simulink model "semi_solarwind"  (R2023b)
settings: Solver=VariableStepAuto  StartTime=0.0  StopTime=5  RelTol=1e-3
undefined symbols (not defined in the file): D1, Delta, Ion, Lithium
libraries: spsSeriesRLCBranchLib x26, spsVoltageMeasurementLib x9, spsDiodeLib x8, dspsrcs4 x8, spsCurrentMeasurementLib x5, spsThreePhaseVIMeasurementLib x5, spsMosfetLib x4, spsPWMGeneratorDCDCLib x4, spsPVArrayLib x4, spsThreePhaseTransformerTwoWindingsLib x3, spsThreePhaseParallelRLCLoadLib x3, spsThreePhaseSeriesRLCBranchLib x3
(part 2 of 2)

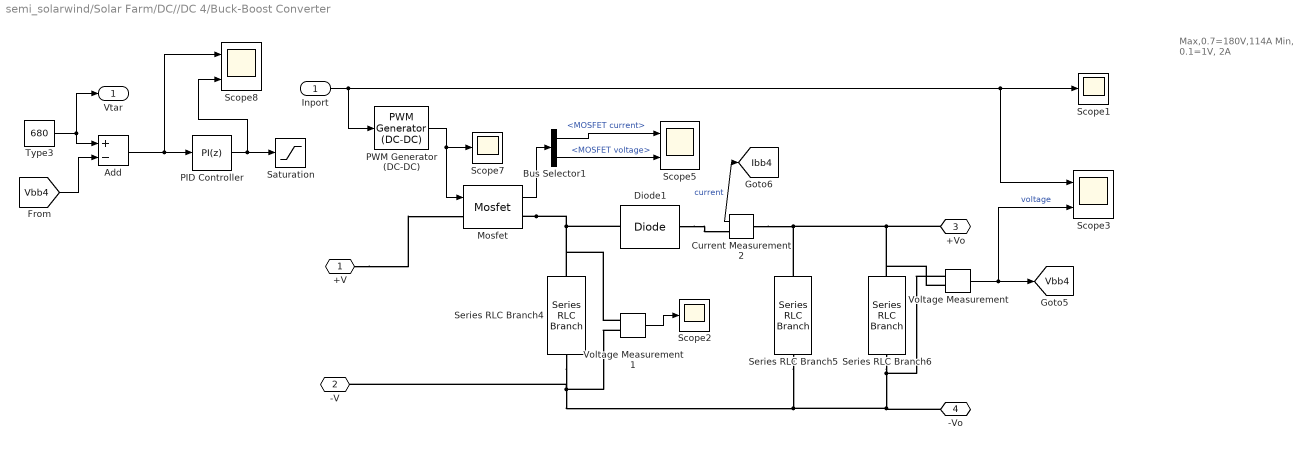
== system semi_solarwind/Solar Farm/DC//DC 4/Buck-Boost Converter ==
  note: Max,0.7=180V,114A
      | Min, 0.1=1V, 2A
  Inport : Inport
  Add : Sum  Inputs=+-
  Bus Selector1 : BusSelector  OutputSignals=MOSFET current,MOSFET voltage
  Current Measurement2 : spsCurrentMeasurementLib/Current Measurement  PhasorSimulation=off  OutputType=Complex  PSBequivalent=0
  Diode1 : spsDiodeLib/Diode  Ron=0.001  Lon=0  Vf=0.8  IC=0  UseSnubber=0  Rs=500  Cs=250e-9  Measurements=off
  Mosfet : spsMosfetLib/Mosfet  Ron=0.1  Lon=0  Rd=0.01  Vfd=0  IC=0  Rs=1e5  Cs=inf  Measurements=on
  PID Controller : slpidlib/PID Controller  Controller=PI  Form=Parallel  TimeDomain=Discrete-time  UseExternalTs=off  SampleTime=-1  IntegratorMethod=Forward Euler  FilterMethod=Forward Euler  ControllerParametersSource=internal  P=0.448206848938492  I=8.01083955194228  UseKiTs=off  D=0  N=100  UseFilter=on  TunerSelectOption=Transfer Function Based (PID Tuner App)  InitialConditionSource=internal  InitialConditionForIntegrator=0  InitialConditionForFilter=0  DifferentiatorICPrevScaledInput=0  ExternalReset=none  TrackingMode=off  Kt=1  LimitOutput=on  SatLimitsSource=internal  UpperSaturationLimit=0.8  LowerSaturationLimit=0  LinearizeAsGain=off  AntiWindupMode=none  Kb=1  LimitIntegrator=on  UpperIntegratorSaturationLimit=0.8  LowerIntegratorSaturationLimit=0  POutMin=[]  POutMax=[]  IOutMin=[]  IOutMax=[]  DOutMin=[]  DOutMax=[]  NOutMin=[]  NOutMax=[]  SumOutMin=[]  SumOutMax=[]  SaturationOutMin=[]  SaturationOutMax=[]  PParamMin=[]  PParamMax=[]  IParamMin=[]  IParamMax=[]  DParamMin=[]  DParamMax=[]  NParamMin=[]  NParamMax=[]  KbParamMin=[]  KbParamMax=[]  KtParamMin=[]  KtParamMax=[]  KbOutMin=[]  KbOutMax=[]  KtOutMin=[]  KtOutMax=[]  IntegratorOutMin=[]  IntegratorOutMax=[]  FilterOutMin=[]  FilterOutMax=[]  SumI1OutMin=[]  SumI1OutMax=[]  SumI2OutMin=[]  SumI2OutMax=[]  SumI3OutMin=[]  SumI3OutMax=[]  SumI4OutMin=[]  SumI4OutMax=[]  SumDOutMin=[]  SumDOutMax=[]  DifferentiatorOutMin=[]  DifferentiatorOutMax=[]  FilterDiffOutCoefMin=[]  FilterDiffOutCoefMax=[]  ReciprocalOutMin=[]  ReciprocalOutMax=[]  SumDenOutMin=[]  SumDenOutMax=[]  SumNumOutMin=[]  SumNumOutMax=[]  DivideOutMin=[]  DivideOutMax=[]  UdiffTsProdOutMin=[]  UdiffTsProdOutMax=[]  NTsProdOutMin=[]  NTsProdOutMax=[]  UintegralTsProdOutMin=[]  UintegralTsProdOutMax=[]  UngainTsProdOutMin=[]  UngainTsProdOutMax=[]  ClampingZeroOutDataTypeStr=Inherit: Inherit via back propagation  ClampingZeroOutMin=[]  ClampingZeroOutMax=[]  FilterDenConstantOutDataTypeStr=Inherit: Inherit via back propagation  FilterDenConstantOutMin=[]  FilterDenConstantOutMax=[]  PCopyOutDataTypeStr=Inherit: Inherit via back propagation  PCopyOutMin=[]  PCopyOutMax=[]  NCopyOutDataTypeStr=Inherit: Inherit via back propagation  NCopyOutMin=[]  NCopyOutMax=[]  IntegratorContinuousStateAttributes=''  IntegratorStateMustResolveToSignalObject=off  IntegratorRTWStateStorageClass=Auto  FilterContinuousStateAttributes=''  FilterStateMustResolveToSignalObject=off  FilterRTWStateStorageClass=Auto  ParallelPVariant=InternalParameters  IdealPVariant=Disabled  IVariant=InternalParameters  DVariant=Disabled  IntegratorVariant=Discrete  SatVariant=Enabled  AWVariant=Passthrough  PCopyVariant=Disabled  TRVariant=Disabled  FdbkBlocksVariant=Forward  IdealPFdbkVariant=Disabled  SatFdbkVariant=Disabled  DerivativeFilterVariant=Disabled  NVariant=Disabled  NCopyVariant=Disabled_SignalSpec  FilterICVariant=Disabled  IntegratorICVariant=InternalICs  ExternalResetVariant=Disabled  TRSumVariant=Passthrough  SumFdbkVariant=Disabled  SumVariant=Sum_PI  TsampFilterVariant=InternalTs  TsampNgainVariant=Passthrough  TsampIntegralVariant=Disabled_SignalSpec  ExternalSaturationOutDataTypeStr=Inherit: Same as second input
  PWM Generator (DC-DC) : spsPWMGeneratorDCDCLib/PWM Generator (DC-DC)  Fsw=900  Ts=0
  Saturation : Saturate  UpperLimit=0.8  LowerLimit=0
  Scope1 : Scope
  Scope2 : Scope
  Scope3 : Scope  NumInputPorts=2
  Scope5 : Scope  NumInputPorts=2
  Scope7 : Scope
  Scope8 : Scope  NumInputPorts=2
  Series RLC Branch4 : spsSeriesRLCBranchLib/Series RLC Branch  LConnTagsString=__new0  RConnTagsString=__new0  BranchType=L  Resistance=1  Inductance=1e-3  SetiL0=off  InitialCurrent=0  Capacitance=1e-6  Setx0=off  InitialVoltage=0  Measurements=None
  Series RLC Branch5 : spsSeriesRLCBranchLib/Series RLC Branch  LConnTagsString=__new0  RConnTagsString=__new0  BranchType=C  Resistance=1  Inductance=1e-3  SetiL0=off  InitialCurrent=0  Capacitance=1e-2  Setx0=off  InitialVoltage=0  Measurements=None
  Series RLC Branch6 : spsSeriesRLCBranchLib/Series RLC Branch  LConnTagsString=__new0  RConnTagsString=__new0  BranchType=R  Resistance=50  Inductance=1e-3  SetiL0=off  InitialCurrent=0  Capacitance=1e-6  Setx0=off  InitialVoltage=0  Measurements=None
  Type3 : Constant  Value=680  SampleTime=0
  Voltage Measurement : spsVoltageMeasurementLib/Voltage Measurement  PhasorSimulation=off  OutputType=Complex  PSBequivalent=0
  Voltage Measurement1 : spsVoltageMeasurementLib/Voltage Measurement  PhasorSimulation=off  OutputType=Complex  PSBequivalent=0
  +V : PMIOPort  Side=Left
  -V : PMIOPort  Port=2  Side=Left
  +Vo : PMIOPort  Port=3  Side=Right
  -Vo : PMIOPort  Port=4  Side=Right
  Vtar : Outport
  tag scope: Ibb4=global, Vbb4=global
  wires:
  [Vbb4] -> Add/2
  Voltage Measurement/1 -> Scope3/2, [Vbb4]  "voltage"
  Bus Selector1/1 -> Scope5/1  "<MOSFET current>"
  Voltage Measurement1/1 -> Scope2/1
  Bus Selector1/2 -> Scope5/2  "<MOSFET voltage>"
  PID Controller/1 -> Scope8/2, Saturation/1
  Add/1 -> Scope8/1, PID Controller/1
  Current Measurement2/1 -> [Ibb4]  "current"
  Type3/1 -> Vtar/1, Add/1
  PWM Generator (DC-DC)/1 -> Mosfet/1, Scope7/1
  Mosfet/1 -> Bus Selector1/1
  Inport/1 -> PWM Generator (DC-DC)/1, Scope3/1, Scope1/1
  connections:
  Series RLC Branch6/RConn1 -- -Vo/RConn1 -- Series RLC Branch4/RConn1 -- -V/RConn1 -- Voltage Measurement1/LConn2 -- Series RLC Branch5/LConn1 -- Voltage Measurement/LConn1
  Mosfet/RConn1 -- Diode1/RConn1 -- Voltage Measurement1/LConn1 -- Series RLC Branch4/LConn1
  Series RLC Branch5/RConn1 -- +Vo/RConn1 -- Voltage Measurement/LConn2 -- Series RLC Branch6/LConn1 -- Current Measurement2/LConn1
  Diode1/LConn1 -- Current Measurement2/RConn1
  +V/RConn1 -- Mosfet/LConn1

== matlab function semi_solarwind/Solar Farm/DC//DC 1/Algorithm ==
  settings: updateMethod=DISCRETE
  data: I input; V input; gpast input; gnext output; duty output; target input; Vbb input
function [gnext, duty] = MPPT(I,V,gpast, target, Vbb)
%% MPPT TESTER FUNCTION
% Select one of the following Perturb & Observe algorithms, by setting Type
% Type=1 for FIXED STEP SIZE
% Type=2 for dP/dV STEP SIZE
% Type=3 for Auto-Scaling
% V input = PV array terminal voltage (V)
% I input = PV array current (A)
%%

duty_init = 0.4;
% min and max value are used to limit duty between
% 0 and 0.85
delta=1e-4; %in steady state
duty_min=0;
duty_max=0.8;


persistent Vpast Ipast Ppast duty_old;
    if isempty(Vpast) % Setup some initial values
        Vpast=0.000001;
        Ipast=0.000001;
        
        %gpast=1;
        duty_old=duty_init;
        Ppast=Vpast*Ipast;
    end


P= V*I; % Measure Power for current iteration 
dI= I - Ipast;
dV= V - Vpast;
dP= P - Ppast;
g=abs(dP);
gpast=abs(gpast);
gup=gpast*1.1;
glow=gpast*0.8;


        if (g>=glow && g<gup)
            delta=delta;   %used to track linear mpp
            
        elseif g>= gup
            %deltaV=3.41*abs(dI*V*(dV/dP));
            delta=(1e-4)*abs(dV*I*(dI/dP));  %used to track curve mpp          
            
        else
            delta=0;
        end



%% MPPT Algorithm  
if dP ~= 0
    if dP < 0
        if dV < 0
            if Vbb < target
                duty=duty_old + delta;
            elseif Vbb > target
                duty=duty_old - delta;
            else
                duty=duty_old;
            end
        else
            if Vbb < target
                duty=duty_old + delta;
            elseif Vbb > target
                duty=duty_old - delta;
            else
                duty=duty_old;
            end
        end
    else
        if dV < 0
            
            if Vbb < target
                duty=duty_old + delta;
            elseif Vbb > target
                duty=duty_old - delta;
            else
                duty=duty_old;
            end
        else
            
            if Vbb < target
                duty=duty_old + delta;
            elseif Vbb > target
                duty=duty_old - delta;
            else
                duty=duty_old;
            end
        end    
    end
else
   
    duty=duty_old;
end


%the below if limits the duty between min and max
if duty > duty_max
    duty=duty_max;
elseif duty<duty_min
    duty=duty_min;
end     

%Pmpp=Vmpp*I;

%%
% Update Past values
duty_old=duty;
Vpast=V;
Ppast=P;
Ipast=I;
gnext = g;
deltaw=delta;
end

== matlab function semi_solarwind/Solar Farm/DC//DC 2/Algorithm ==
  settings: updateMethod=DISCRETE
  data: I input; V input; gpast input; gnext output; duty output; target input; Vbb input
function [gnext, duty] = MPPT(I,V,gpast, target, Vbb)
%% MPPT TESTER FUNCTION
% Select one of the following Perturb & Observe algorithms, by setting Type
% Type=1 for FIXED STEP SIZE
% Type=2 for dP/dV STEP SIZE
% Type=3 for Auto-Scaling
% V input = PV array terminal voltage (V)
% I input = PV array current (A)
%%

duty_init = 0.4;
% min and max value are used to limit duty between
% 0 and 0.85
delta=1e-4; %in steady state
duty_min=0;
duty_max=0.8;


persistent Vpast Ipast Ppast duty_old;
    if isempty(Vpast) % Setup some initial values
        Vpast=0.000001;
        Ipast=0.000001;
        
        %gpast=1;
        duty_old=duty_init;
        Ppast=Vpast*Ipast;
    end


P= V*I; % Measure Power for current iteration 
dI= I - Ipast;
dV= V - Vpast;
dP= P - Ppast;
g=abs(dP);
gpast=abs(gpast);
gup=gpast*1.1;
glow=gpast*0.8;


        if (g>=glow && g<gup)
            delta=delta;   %used to track linear mpp
            
        elseif g>= gup
            %deltaV=3.41*abs(dI*V*(dV/dP));
            delta=(1e-4)*abs(dV*I*(dI/dP));  %used to track curve mpp          
            
        else
            delta=0;
        end



%% MPPT Algorithm  
if dP ~= 0
    if dP < 0
        if dV < 0
            if Vbb < target
                duty=duty_old + delta;
            elseif Vbb > target
                duty=duty_old - delta;
            else
                duty=duty_old;
            end
        else
            if Vbb < target
                duty=duty_old + delta;
            elseif Vbb > target
                duty=duty_old - delta;
            else
                duty=duty_old;
            end
        end
    else
        if dV < 0
            
            if Vbb < target
                duty=duty_old + delta;
            elseif Vbb > target
                duty=duty_old - delta;
            else
                duty=duty_old;
            end
        else
            
            if Vbb < target
                duty=duty_old + delta;
            elseif Vbb > target
                duty=duty_old - delta;
            else
                duty=duty_old;
            end
        end    
    end
else
   
    duty=duty_old;
end


%the below if limits the duty between min and max
if duty > duty_max
    duty=duty_max;
elseif duty<duty_min
    duty=duty_min;
end     

%Pmpp=Vmpp*I;

%%
% Update Past values
duty_old=duty;
Vpast=V;
Ppast=P;
Ipast=I;
gnext = g;
deltaw=delta;
end

== matlab function semi_solarwind/Solar Farm/DC//DC 3/Algorithm ==
  settings: updateMethod=DISCRETE
  data: I input; V input; gpast input; gnext output; duty output; target input; Vbb input
function [gnext, duty] = MPPT(I,V,gpast, target, Vbb)
%% MPPT TESTER FUNCTION
% Select one of the following Perturb & Observe algorithms, by setting Type
% Type=1 for FIXED STEP SIZE
% Type=2 for dP/dV STEP SIZE
% Type=3 for Auto-Scaling
% V input = PV array terminal voltage (V)
% I input = PV array current (A)
%%

duty_init = 0.4;
% min and max value are used to limit duty between
% 0 and 0.85
delta=1e-4; %in steady state
duty_min=0;
duty_max=0.8;


persistent Vpast Ipast Ppast duty_old;
    if isempty(Vpast) % Setup some initial values
        Vpast=0.000001;
        Ipast=0.000001;
        
        %gpast=1;
        duty_old=duty_init;
        Ppast=Vpast*Ipast;
    end


P= V*I; % Measure Power for current iteration 
dI= I - Ipast;
dV= V - Vpast;
dP= P - Ppast;
g=abs(dP);
gpast=abs(gpast);
gup=gpast*1.1;
glow=gpast*0.8;


        if (g>=glow && g<gup)
            delta=delta;   %used to track linear mpp
            
        elseif g>= gup
            %deltaV=3.41*abs(dI*V*(dV/dP));
            delta=(1e-4)*abs(dV*I*(dI/dP));  %used to track curve mpp          
            
        else
            delta=0;
        end



%% MPPT Algorithm  
if dP ~= 0
    if dP < 0
        if dV < 0
            if Vbb < target
                duty=duty_old + delta;
            elseif Vbb > target
                duty=duty_old - delta;
            else
                duty=duty_old;
            end
        else
            if Vbb < target
                duty=duty_old + delta;
            elseif Vbb > target
                duty=duty_old - delta;
            else
                duty=duty_old;
            end
        end
    else
        if dV < 0
            
            if Vbb < target
                duty=duty_old + delta;
            elseif Vbb > target
                duty=duty_old - delta;
            else
                duty=duty_old;
            end
        else
            
            if Vbb < target
                duty=duty_old + delta;
            elseif Vbb > target
                duty=duty_old - delta;
            else
                duty=duty_old;
            end
        end    
    end
else
   
    duty=duty_old;
end


%the below if limits the duty between min and max
if duty > duty_max
    duty=duty_max;
elseif duty<duty_min
    duty=duty_min;
end     

%Pmpp=Vmpp*I;

%%
% Update Past values
duty_old=duty;
Vpast=V;
Ppast=P;
Ipast=I;
gnext = g;
deltaw=delta;
end

== matlab function semi_solarwind/Solar Farm/DC//DC 4/Algorithm ==
  settings: updateMethod=DISCRETE
  data: I input; V input; gpast input; gnext output; duty output; target input; Vbb input
function [gnext, duty] = MPPT(I,V,gpast, target, Vbb)
%% MPPT TESTER FUNCTION
% Select one of the following Perturb & Observe algorithms, by setting Type
% Type=1 for FIXED STEP SIZE
% Type=2 for dP/dV STEP SIZE
% Type=3 for Auto-Scaling
% V input = PV array terminal voltage (V)
% I input = PV array current (A)
%%

duty_init = 0.4;
% min and max value are used to limit duty between
% 0 and 0.85
delta=1e-4; %in steady state
duty_min=0;
duty_max=0.8;


persistent Vpast Ipast Ppast duty_old;
    if isempty(Vpast) % Setup some initial values
        Vpast=0.000001;
        Ipast=0.000001;
        
        %gpast=1;
        duty_old=duty_init;
        Ppast=Vpast*Ipast;
    end


P= V*I; % Measure Power for current iteration 
dI= I - Ipast;
dV= V - Vpast;
dP= P - Ppast;
g=abs(dP);
gpast=abs(gpast);
gup=gpast*1.1;
glow=gpast*0.8;


        if (g>=glow && g<gup)
            delta=delta;   %used to track linear mpp
            
        elseif g>= gup
            %deltaV=3.41*abs(dI*V*(dV/dP));
            delta=(1e-4)*abs(dV*I*(dI/dP));  %used to track curve mpp          
            
        else
            delta=0;
        end



%% MPPT Algorithm  
if dP ~= 0
    if dP < 0
        if dV < 0
            if Vbb < target
                duty=duty_old + delta;
            elseif Vbb > target
                duty=duty_old - delta;
            else
                duty=duty_old;
            end
        else
            if Vbb < target
                duty=duty_old + delta;
            elseif Vbb > target
                duty=duty_old - delta;
            else
                duty=duty_old;
            end
        end
    else
        if dV < 0
            
            if Vbb < target
                duty=duty_old + delta;
            elseif Vbb > target
                duty=duty_old - delta;
            else
                duty=duty_old;
            end
        else
            
            if Vbb < target
                duty=duty_old + delta;
            elseif Vbb > target
                duty=duty_old - delta;
            else
                duty=duty_old;
            end
        end    
    end
else
   
    duty=duty_old;
end


%the below if limits the duty between min and max
if duty > duty_max
    duty=duty_max;
elseif duty<duty_min
    duty=duty_min;
end     

%Pmpp=Vmpp*I;

%%
% Update Past values
duty_old=duty;
Vpast=V;
Ppast=P;
Ipast=I;
gnext = g;
deltaw=delta;
end
